simulink model "Sim_partie1_bis"  (R2023b)
settings: Solver=FixedStepAuto  StartTime=0.0  StopTime=1000000  FixedStep=10  RelTol=1e-3
undefined symbols (not defined in the file): G, Mt, phi, r, Rt, theta, v0
libraries: simulink x2
settings Model: Creator=louis  LastModifiedBy=louis

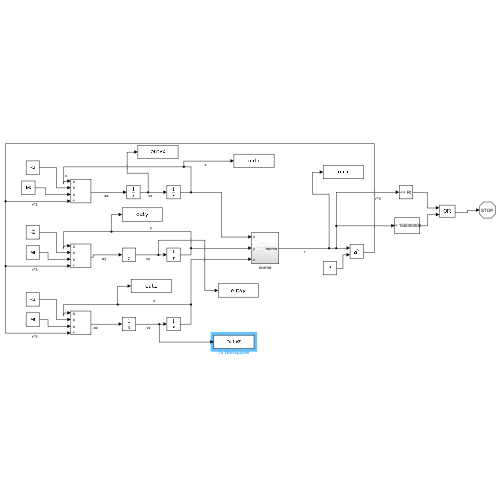
[thumbnail: Simulink's stored preview of the top-level diagram]
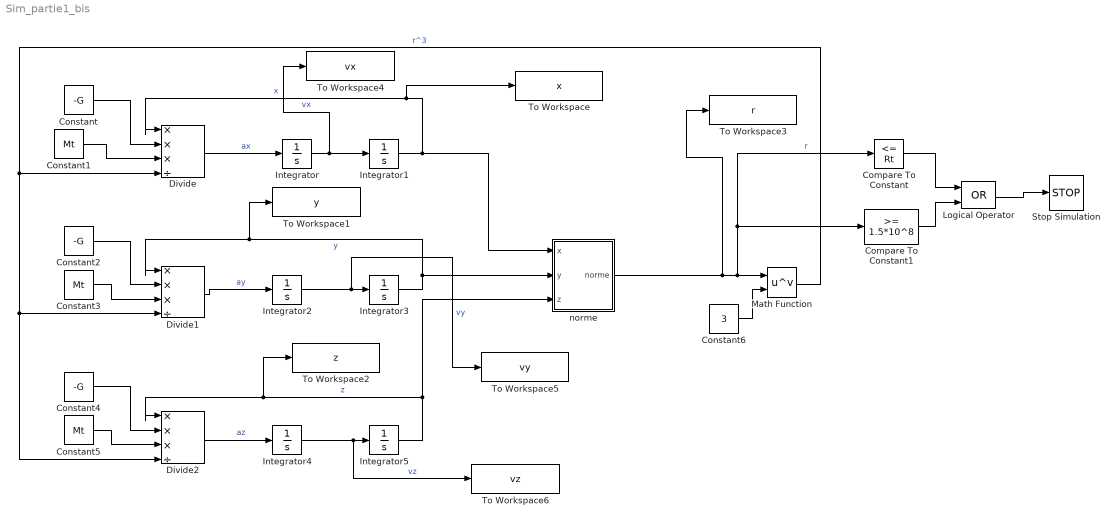
== system Sim_partie1_bis ==
  Compare To Constant : simulink/Logic and Bit Operations/Compare To Constant  relop=<=  const=Rt  OutDataTypeStr=boolean
  Compare To Constant1 : simulink/Logic and Bit Operations/Compare To Constant  relop=>=  const=1.5*10^8  OutDataTypeStr=boolean
  Constant : Constant  Value=-G
  Constant1 : Constant  Value=Mt
  Constant2 : Constant  Value=-G
  Constant3 : Constant  Value=Mt
  Constant4 : Constant  Value=-G
  Constant5 : Constant  Value=Mt
  Constant6 : Constant  Value=3
  Divide : Product  Inputs=***/
  Divide1 : Product  Inputs=***/
  Divide2 : Product  Inputs=***/
  Integrator : Integrator  InitialCondition=v0*sind(theta)
  Integrator1 : Integrator  InitialCondition=r*sind(phi)*cosd(theta)
  Integrator2 : Integrator  InitialCondition=-v0*cosd(theta)
  Integrator3 : Integrator  InitialCondition=r*sind(phi)*sind(theta)
  Integrator4 : Integrator
  Integrator5 : Integrator  InitialCondition=r*cosd(phi)
  Logical Operator : Logic  Operator=OR  AllPortsSameDT=off  OutDataTypeStr=boolean
  Math Function : Math  Operator=pow
  Stop Simulation : Stop
  To Workspace : ToWorkspace  VariableName=x  SaveFormat=Timeseries  SampleTime=-1
  To Workspace1 : ToWorkspace  VariableName=y  SaveFormat=Timeseries  SampleTime=-1
  To Workspace2 : ToWorkspace  VariableName=z  SaveFormat=Timeseries  SampleTime=-1
  To Workspace3 : ToWorkspace  VariableName=r  SaveFormat=Timeseries  SampleTime=-1
  To Workspace4 : ToWorkspace  VariableName=vx  SaveFormat=Timeseries  SampleTime=-1
  To Workspace5 : ToWorkspace  VariableName=vy  SaveFormat=Timeseries  SampleTime=-1
  To Workspace6 : ToWorkspace  VariableName=vz  SaveFormat=Timeseries  SampleTime=-1
  norme : Subsystem
  wires:
  Constant/1 -> Divide/2
  Constant1/1 -> Divide/3
  Divide/1 -> Integrator/1  "ax"
  Integrator/1 -> To Workspace4/1, Integrator1/1  "vx"
  Integrator1/1 -> norme/1(x), To Workspace/1, Divide/1  "x"
  Integrator3/1 -> To Workspace1/1, Divide1/1, norme/2(y)  "y"
  Integrator2/1 -> To Workspace5/1, Integrator3/1  "vy"
  Constant2/1 -> Divide1/2
  Constant3/1 -> Divide1/3
  Divide1/1 -> Integrator2/1  "ay"
  Integrator5/1 -> norme/3(z), To Workspace2/1, Divide2/1  "z"
  Integrator4/1 -> To Workspace6/1, Integrator5/1  "vz"
  Constant4/1 -> Divide2/2
  Constant5/1 -> Divide2/3
  Divide2/1 -> Integrator4/1  "az"
  Constant6/1 -> Math Function/2
  Math Function/1 -> Divide2/4, Divide1/4, Divide/4  "r^3"
  Compare To Constant1/1 -> Logical Operator/2
  Compare To Constant/1 -> Logical Operator/1
  Logical Operator/1 -> Stop Simulation/1
  norme/1(norme) -> To Workspace3/1, Compare To Constant1/1, Compare To Constant/1, Math Function/1  "r"

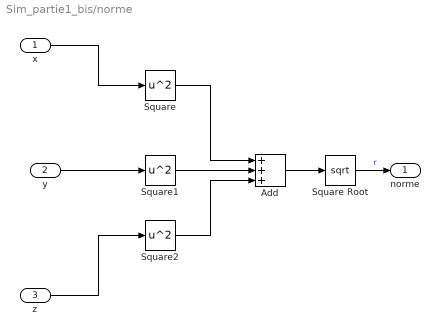
== system Sim_partie1_bis/norme ==
  x : Inport
  y : Inport  Port=2
  z : Inport  Port=3
  Add : Sum  Inputs=+++
  Square : Math  Operator=square
  Square Root : Sqrt
  Square1 : Math  Operator=square
  Square2 : Math  Operator=square
  norme : Outport
  wires:
  Add/1 -> Square Root/1
  x/1 -> Square/1
  Square2/1 -> Add/3
  Square1/1 -> Add/2
  Square/1 -> Add/1
  y/1 -> Square1/1
  z/1 -> Square2/1
  Square Root/1 -> norme/1  "r"
